simulink model "DSP_Project_Simulink"  (R2023b)
settings: Solver=FixedStepDiscrete  StartTime=0.0  StopTime=inf  RelTol=1e-3  EnableMultiTasking=on
libraries: dspvision x4, dspindex x2, dspsrcs4 x2, dspsnks4 x2, dspadpt3 x2, dspobslib x2
settings Model: Creator=The MathWorks, Inc.  LastModifiedBy=abhin
settings SolverCC: AlgebraicLoopSolver=TrustRegion  MaxZcPerStep=1
settings DataIOCC: SaveFormat=Array  SaveOutput=off  SaveTime=off  ReturnWorkspaceOutputs=off  SignalLoggingName=sigsOut
settings OptimizationCC: ExpressionDepthLimit=2147483647  InitFltsAndDblsToZero=on  EfficientMapNaN2IntZero=off  LifeSpan=inf  SimCompilerOptimization=on
settings DebuggingCC: UnderspecifiedInitializationDetection=Classic  MergeDetectMultiDrivingBlocksExec=none  CheckExecutionContextPreStartOutputMsg=on  SignalResolutionControl=TryResolveAllWithWarning  MultiTaskDSMMsg=warning  MultiTaskCondExecSysMsg=none  ParameterPrecisionLossMsg=none  FcnCallInpInsideContextMsg=warning  UnconnectedInputMsg=warning  UnconnectedOutputMsg=warning  UnconnectedLineMsg=warning  AllowSymbolicDim=off  StateNameClashWarn=warning  SymbolicDimsDataTypeCodeGenerationDiagnostic=none  SFUnexpectedBacktrackingDiag=warning  SFNoUnconditionalDefaultTransitionDiag=warning  SFExecutionAtInitializationDiag=none  ArithmeticOperatorsInVariantConditions=warning
settings HardwareCC: ProdBitPerPointer=32  ProdBitPerSizeT=32  ProdBitPerPtrDiffT=32  ProdLargestAtomicFloat=None  ProdIntDivRoundTo=Undefined  ProdEndianess=Unspecified  ProdWordSize=32  ProdHWDeviceType=32-bit Generic  TargetUnknown=on
settings ModelReferenceCC: UpdateModelReferenceTargets=IfOutOfDate  EnableRefExpFcnMdlSchedulingChecks=on  PropagateSignalLabelsOutOfModel=off
settings SFSimCC: SimUseLocalCustomCode=off  CustomCodeUndefinedFunction=UseInterfaceOnly
settings RTWCC: RTWUseLocalCustomCode=off  DLArmComputeVersion=19.05
settings CodeAppCC: StateflowObjectComments=on
settings GRTTargetCC: TargetFcnLib=ansi_tfl_tmw_new.mat  TargetLangStandard=C89/C90 (ANSI)  CombineOutputUpdateFcns=off  GRTInterface=on
settings ConfigComp: CovMetricSettings=dw  CovSaveCumulativeToWorkspaceVar=on  CovSaveSingleToWorkspaceVar=on  CovExternalEMLEnable=off  CovSFcnEnable=off

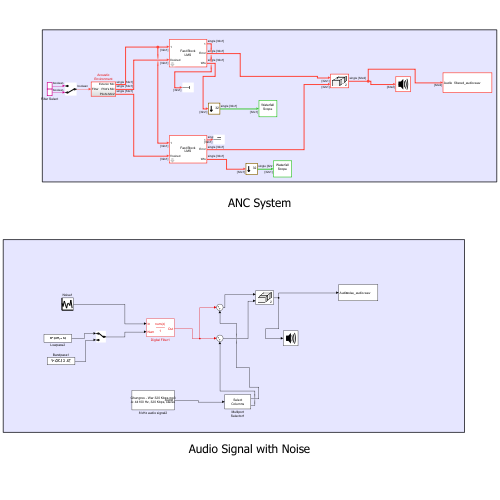
[thumbnail: Simulink's stored preview of the top-level diagram]
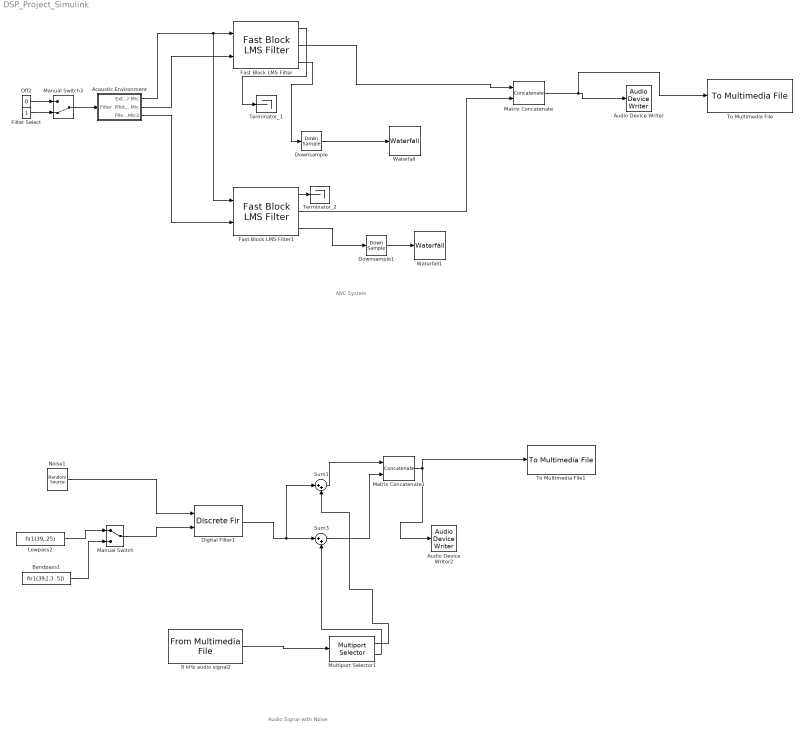
== system DSP_Project_Simulink ==
  note: ANC System
  note: Audio Signal with Noise
  8 kHz audio signal2 : dspvision/From Multimedia File  inputFilename=C:\Users\abhin\Downloads\Ghungroo - War 320 Kbps.mp3  readRange=[1 Inf]  loop=on  numPlays=inf  outputStreams=Audio only  videoDataType=single  audioDataType=single  inheritSampleTime=on  userDefinedSampleTime=1/30  noAudioOutput=off  isIntensityVideo=off  fourcc=RGB  colorVideoFormat=Separate color signals  outputEOF=off  dataOrg=Column-major  audioFrameSize=32  computeAudioFrameSize=off  outSamplingMode=Sample based
  Acoustic Environment : Subsystem
  Audio Device Writer : dspsnks4/Audio Device Writer  Driver=DirectSound  Device=AI Noise-cancelling Output (ASUS Utility)  InheritSampleRate=on  SampleRate=44100  BitDepth=16-bit integer  BufferSize=4096  NumBuffers=10  DefaultOutputChannelMapping=on  OutputChannelMapping=1:2  OutputNumUnderrunSamples=off  DriverIdx=1  DeviceWarnFlag=''
  Audio Device Writer2 : dspsnks4/Audio Device Writer  Driver=DirectSound  Device=AI Noise-cancelling Output (ASUS Utility)  InheritSampleRate=on  SampleRate=44100  BitDepth=16-bit integer  BufferSize=4096  NumBuffers=10  DefaultOutputChannelMapping=on  OutputChannelMapping=1:2  OutputNumUnderrunSamples=off  DriverIdx=1  DeviceWarnFlag=''
  Bandpass1 : Constant  Value=fir1(39,[.3 .5])  OutDataTypeStr=Inherit: Inherit via back propagation
  Digital Filter1 : DiscreteFir  CoefSource=Input port  Coefficients=[1 2]  InputProcessing=Columns as channels (frame based)  AccumDataTypeStr=Inherit: Same as product output  OutDataTypeStr=Inherit: Same as input
      settings: InputPortMap=u0,u1
  Downsample : DownSample  N=32  RateOptions=Allow multirate processing
  Downsample1 : DownSample  N=32  RateOptions=Allow multirate processing
  Fast Block LMS Filter : dspadpt3/Fast Block LMS Filter  algo=Fast Block LMS  L=32  N=32  stepflag=Dialog  mu=0.0005  leakage=1.0  addnparflag=on  ic=0  Adapt=off  resetflag=None  weights=on
  Fast Block LMS Filter1 : dspadpt3/Fast Block LMS Filter  algo=Fast Block LMS  L=32  N=32  stepflag=Dialog  mu=0.0005  leakage=1.0  addnparflag=on  ic=0  Adapt=off  resetflag=None  weights=on
  Filter Select : Constant  OutDataTypeStr=boolean
  Lowpass2 : Constant  Value=fir1(39,.25)  OutDataTypeStr=Inherit: Inherit via back propagation
  Manual Switch : ManualSwitch
  Manual Switch3 : ManualSwitch  CurrentSetting=0
  Matrix Concatenate : Concatenate  Mode=Multidimensional array  ConcatenateDimension=2
  Matrix Concatenate1 : Concatenate  Mode=Multidimensional array  ConcatenateDimension=2
  Multiport Selector1 : dspindex/Multiport Selector  rowsOrCols=Columns  idxCellArray={1,2}  idxErrMode=Clip Index
      settings: LibrarySourceBlock=|
      | dsphdlsupportsigmgmt/Multiport
      | Selector
  Noise1 : dspsrcs4/Random Source  SrcType=Gaussian  NormMethod=Sum of uniform values  CltLength=5  MinVal=-1  MaxVal=1  MeanVal=0  VarVal=1  RepMode=Specify seed  rawSeed=[23341]  IsInherit=off  SampMode=Discrete  SampTime=1/44100  SampFrame=32  DataType=Single  OutComplex=Real  OutputFrames=off
  Off2 : Constant  Value=0  OutDataTypeStr=boolean
  Sum1 : Sum  Inputs=|++  InputSameDT=on  SaturateOnIntegerOverflow=on  OutDataTypeStr=Inherit: Same as first input
  Sum3 : Sum  Inputs=|++  InputSameDT=on  SaturateOnIntegerOverflow=on  OutDataTypeStr=Inherit: Same as first input
  Terminator_1 : Terminator
  Terminator_2 : Terminator
  To Multimedia File : dspvision/To Multimedia File  outputFilename=filtered_audio.wav  streamSelection=Audio only  videoCompressor=None (uncompressed)  audioCompressor=None (uncompressed)  imagePorts=One multidimensional signal  fileType=WAV  audioDatatype=16-bit integer  fourcc=RGB  videoQuality=75  mj2000CompFactor=10
      settings: LibrarySourceBlock=dspsnks4/To Multimedia File
  To Multimedia File1 : dspvision/To Multimedia File  outputFilename=noise_audio.wav  streamSelection=Audio only  videoCompressor=None (uncompressed)  audioCompressor=None (uncompressed)  imagePorts=One multidimensional signal  fileType=WAV  audioDatatype=16-bit integer  fourcc=RGB  videoQuality=75  mj2000CompFactor=10
      settings: LibrarySourceBlock=dspsnks4/To Multimedia File
  Waterfall : dspobslib/Waterfall  TraceProperties=off  NumTraces=6  CMapStr=autumn  TNewest=0.9  TOldest=0.5  HistoryLength=50  HistoryFull=Overwrite  UpdateInterval=1  ExportMode=All visible  MLExportName=ExportData  AutoExport=off  DisplayProperties=on  MouseMode=Orbit  AxisGrid=on  Snapshot=off  Suspend=off  SyncSnapshots=off  OpenScopeAtSimStart=on  FigPos=[618.333333333333 133.666666666667 405.333333333333 338.666666666667]  CameraView=[28.5695107359948 1316.8235109177 -294.350451091202 -0.004386576265097 22.5 3.5 0.594111941595966 -49.3321641526923 11.3523452384532 1.20078102376266 1 86.3856203154502 14.008478970073]  InportDimsHint=[32 1]  AxisProperties=off  AxisColor='w'  XLabel=Samples  YLabel=Amplitude  ZLabel=Time  TriggerProperties=off  TrigStartMode=Immediately  TrigStartT=0  TrigStartN=0  TrigStartFcn=trigbegin  TrigStopMode=Never  TrigStopT=0.1  TrigStopN=1  TrigStopFcn=trigend  TrigRearmMode=Never  TrigRearmT=0  TrigRearmN=0  TrigRearmFcn=trigrearm  XformProperties=off  XformMode=None  XformFcn=abs  XformExpr=(u+1)/2
      settings: YMin=-0.188312025368214  YMax=0.24
  Waterfall1 : dspobslib/Waterfall  TraceProperties=off  NumTraces=6  CMapStr=autumn  TNewest=0.9  TOldest=0.5  HistoryLength=50  HistoryFull=Overwrite  UpdateInterval=1  ExportMode=All visible  MLExportName=ExportData  AutoExport=off  DisplayProperties=on  MouseMode=Orbit  AxisGrid=on  Snapshot=off  Suspend=off  SyncSnapshots=off  OpenScopeAtSimStart=on  FigPos=[618.333333333333 133.666666666667 405.333333333333 338.666666666667]  CameraView=[28.5695107359948 1316.8235109177 -294.350451091202 -0.004386576265097 22.5 3.5 0.594111941595966 -49.3321641526923 11.3523452384532 1.20078102376266 1 86.3856203154502 14.008478970073]  InportDimsHint=[32 1]  AxisProperties=off  AxisColor='w'  XLabel=Samples  YLabel=Amplitude  ZLabel=Time  TriggerProperties=off  TrigStartMode=Immediately  TrigStartT=0  TrigStartN=0  TrigStartFcn=trigbegin  TrigStopMode=Never  TrigStopT=0.1  TrigStopN=1  TrigStopFcn=trigend  TrigRearmMode=Never  TrigRearmT=0  TrigRearmN=0  TrigRearmFcn=trigrearm  XformProperties=off  XformMode=None  XformFcn=abs  XformExpr=(u+1)/2
      settings: YMin=-0.188312025368214  YMax=0.24
  wires:
  Acoustic Environment/2(Pilot's Mic) -> Fast Block LMS Filter/2
  Off2/1 -> Manual Switch3/1
  Filter Select/1 -> Manual Switch3/2
  Manual Switch3/1 -> Acoustic Environment/1(Filter)
  Fast Block LMS Filter/1 -> Terminator_1/1
  Fast Block LMS Filter/2 -> Matrix Concatenate/1
  Fast Block LMS Filter/3 -> Downsample/1
  Downsample/1 -> Waterfall/1
  Acoustic Environment/3(Pilot's Mic2) -> Fast Block LMS Filter1/2
  Fast Block LMS Filter1/2 -> Matrix Concatenate/2
  Fast Block LMS Filter1/3 -> Downsample1/1
  Downsample1/1 -> Waterfall1/1
  Fast Block LMS Filter1/1 -> Terminator_2/1
  Acoustic Environment/1(Exterior Mic) -> Fast Block LMS Filter1/1, Fast Block LMS Filter/1
  Matrix Concatenate/1 -> To Multimedia File/1, Audio Device Writer/1
  Multiport Selector1/2 -> Sum3/2
  Manual Switch/1 -> Digital Filter1/2
  Sum3/1 -> Matrix Concatenate1/2
  Multiport Selector1/1 -> Sum1/2
  Digital Filter1/1 -> Sum1/1, Sum3/1
  Noise1/1 -> Digital Filter1/1
  Bandpass1/1 -> Manual Switch/2
  Lowpass2/1 -> Manual Switch/1
  8 kHz audio signal2/1 -> Multiport Selector1/1
  Sum1/1 -> Matrix Concatenate1/1
  Matrix Concatenate1/1 -> Audio Device Writer2/1, To Multimedia File1/1

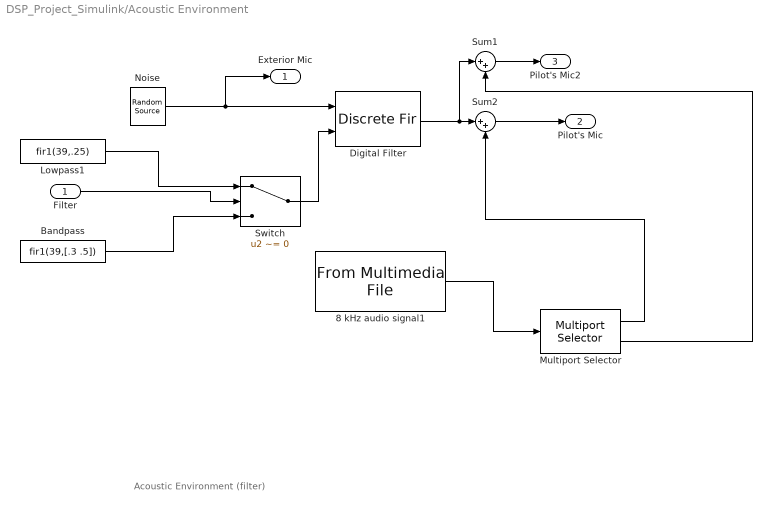
== system DSP_Project_Simulink/Acoustic Environment ==
  note: Acoustic Environment (filter)
  Filter : Inport
  8 kHz audio signal1 : dspvision/From Multimedia File  inputFilename=C:\Users\abhin\Downloads\Alan-Walker-Sabrina-Carpenter-Farruko-On-My-Way.mp3  readRange=[1 Inf]  loop=on  numPlays=inf  outputStreams=Audio only  videoDataType=single  audioDataType=single  inheritSampleTime=on  userDefinedSampleTime=1/30  noAudioOutput=off  isIntensityVideo=off  fourcc=RGB  colorVideoFormat=Separate color signals  outputEOF=off  dataOrg=Column-major  audioFrameSize=32  computeAudioFrameSize=off  outSamplingMode=Sample based
  Bandpass : Constant  Value=fir1(39,[.3 .5])  OutDataTypeStr=Inherit: Inherit via back propagation
  Digital Filter : DiscreteFir  CoefSource=Input port  Coefficients=[1 2]  InputProcessing=Columns as channels (frame based)  AccumDataTypeStr=Inherit: Same as product output  OutDataTypeStr=Inherit: Same as input
      settings: InputPortMap=u0,u1
  Lowpass1 : Constant  Value=fir1(39,.25)  OutDataTypeStr=Inherit: Inherit via back propagation
  Multiport Selector : dspindex/Multiport Selector  rowsOrCols=Columns  idxCellArray={1,2}  idxErrMode=Clip Index
      settings: LibrarySourceBlock=|
      | dsphdlsupportsigmgmt/Multiport
      | Selector
  Noise : dspsrcs4/Random Source  SrcType=Gaussian  NormMethod=Sum of uniform values  CltLength=5  MinVal=-1  MaxVal=1  MeanVal=0  VarVal=1  RepMode=Specify seed  rawSeed=[23341]  IsInherit=off  SampMode=Discrete  SampTime=1/44100  SampFrame=32  DataType=Single  OutComplex=Real  OutputFrames=off
  Sum1 : Sum  Inputs=|++  InputSameDT=on  SaturateOnIntegerOverflow=on  OutDataTypeStr=Inherit: Same as first input
  Sum2 : Sum  Inputs=|++  InputSameDT=on  SaturateOnIntegerOverflow=on  OutDataTypeStr=Inherit: Same as first input
  Switch : Switch  Criteria=u2 ~= 0  InputSameDT=off
  Exterior Mic : Outport  VectorParamsAs1DForOutWhenUnconnected=off
  Pilot's Mic : Outport  Port=2  VectorParamsAs1DForOutWhenUnconnected=off
  Pilot's Mic2 : Outport  Port=3  VectorParamsAs1DForOutWhenUnconnected=off
  wires:
  8 kHz audio signal1/1 -> Multiport Selector/1
  Sum2/1 -> Pilot's Mic/1
  Filter/1 -> Switch/2
  Digital Filter/1 -> Sum1/1, Sum2/1
  Noise/1 -> Digital Filter/1, Exterior Mic/1
  Switch/1 -> Digital Filter/2
  Bandpass/1 -> Switch/3
  Lowpass1/1 -> Switch/1
  Multiport Selector/1 -> Sum2/2
  Multiport Selector/2 -> Sum1/2
  Sum1/1 -> Pilot's Mic2/1
